simulink model "Plant"  (R2025b)
settings: Solver=VariableStepAuto  StartTime=0.0  StopTime=10.0  RelTol=1e-3
values from neighbouring files (symbols this model uses):
  eul_init = scenario.eul_init    [Brown_6DOF_Init_main.m]    (also in Full_Sim_Init.m; Run_Main.m = runSpec.eul_init)
  g = scenario.g    [Brown_6DOF_Init_main.m]    (also in Full_Sim_Init.m; aircraft_def.m = value)
  J = aircraft.J    [Brown_6DOF_Init_main.m]    (also in Full_Sim_Init.m; HOMEWORK7_trim_linmod_live_source.m = zeros(4,3); aircraft_def.m = I_total)
  Mass = aircraft.Mass    [Brown_6DOF_Init_main.m]    (also in Full_Sim_Init.m; aircraft_def.m = 0)
  omega_init = scenario.omega_init    [Brown_6DOF_Init_main.m]    (also in Full_Sim_Init.m; Run_Main.m = runSpec.omega_init)
  pos_init = scenario.pos_init    [Brown_6DOF_Init_main.m]    (also in Full_Sim_Init.m; Run_Main.m = runSpec.pos_init)
  prop = aircraft.prop    [Brown_6DOF_Init_main.m]    (also in Full_Sim_Init.m; Run_INDI_Qdot_Effectiveness_Audit.m = plant.prop)
  q = q / norm(q)    [HOMEWORK7_trim_linmod_live_source.m]    (also in attitude_complementary_step.m = gyro_meas(2))
  r = positions(i, :).'-cg(:)    [Run_INDI_Qdot_Effectiveness_Audit.m]    (also in attitude_complementary_step.m = gyro_meas(3))
  V_init = scenario.V_init    [Brown_6DOF_Init_main.m]    (also in Full_Sim_Init.m; Run_Main.m = runSpec.V_init)
undefined symbols (not defined in the file or in its folder): F, Light, magnitude, MIL
libraries: eVTOL_lib x23, aerolibwind2 x1
settings Model: Creator=zbrown  LastModifiedBy=zbrown

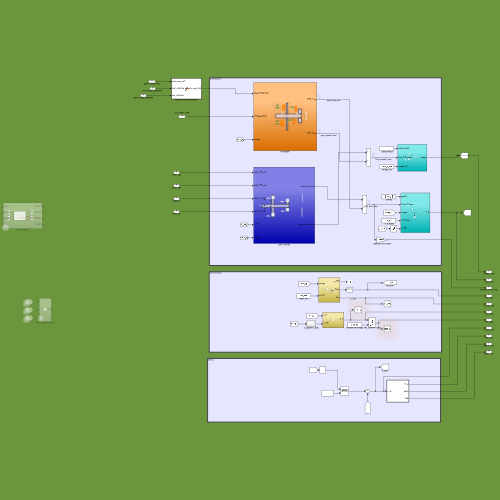
[thumbnail: Simulink's stored preview of the top-level diagram]
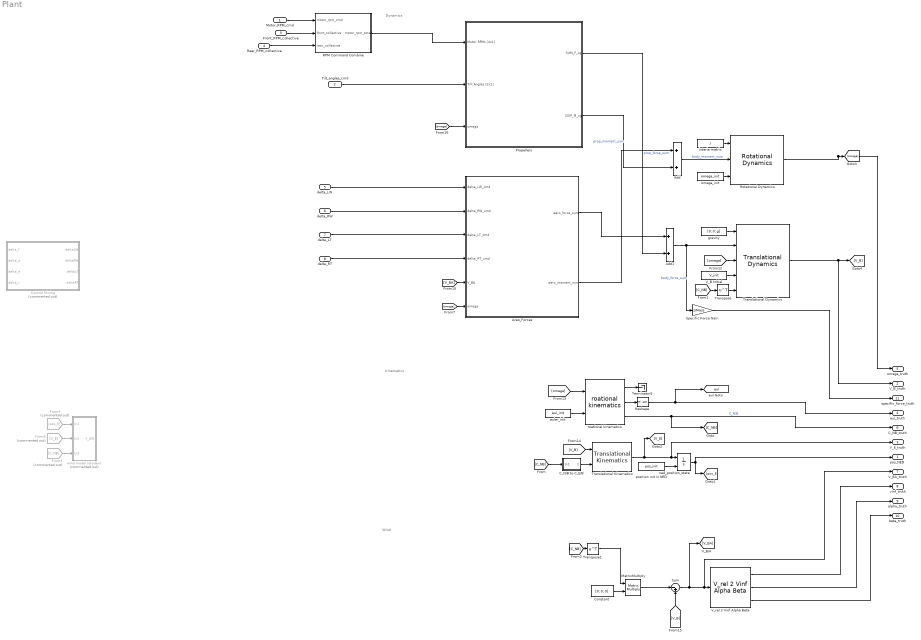
== system Plant ==
  note: Wind
  note: Dynamics
  note: Kinematics
  Motor_RPM_cmd : Inport  PortDimensions=4
  Tilt_angles_cmd : Inport  Port=2  PortDimensions=2
  Front_RPM_collective : Inport  Port=3
  Rear_RPM_collective : Inport  Port=4
  delta_LW : Inport  Port=5
  delta_RW : Inport  Port=6
  delta_LT : Inport  Port=7
  delta_RT : Inport  Port=8
  " V_B Initial" : Constant  Value=V_init
  " gravity" : Constant  Value=[0; 0; g]
  " interia matrix" : Constant  Value=J
  Add : Sum
  Add1 : Sum
  Areo_Forces : Subsystem
  C_N/B to C_E/B : Subsystem
  Constant : Constant  Value=[0; 0; 0]
  Control Mixing : Subsystem  Commented=on
  From3 : From  Commented=on  GotoTag=C_NB
  From4 : From  Commented=on  GotoTag=pos_E
  From5 : From  Commented=on  GotoTag=V_E
  MatrixMultiply : Product  Multiplication=Matrix(*)
  Propellers : Subsystem
  RPM Command Combine : MATLAB Function  TreatAsAtomicUnit=on
  Reshape : Reshape
  Rotational Dynamics : eVTOL_lib/Rotational Dynamics  SystemSampleTime=-1  VariantActivationTime=update diagram  EmptyChoice=off  PassThrough=off  PassThroughVariantControl=(default)  EmptyChoiceVariantControl=(default)  AllowFlexibleInterface=on  Latency=0  AutoFrameSizeCalculation=off
  Specific Force Gain : Gain  Gain=1/Mass
  Sum : Sum  Inputs=|-+
  Terminator5 : Terminator
  Translational Dynamics : eVTOL_lib/Translational Dynamics  SystemSampleTime=-1  VariantActivationTime=update diagram  EmptyChoice=off  PassThrough=off  PassThroughVariantControl=(default)  EmptyChoiceVariantControl=(default)  AllowFlexibleInterface=on  Latency=0  AutoFrameSizeCalculation=off
  Translational Kinematics : eVTOL_lib/Translational Kinematics  SystemSampleTime=-1  VariantActivationTime=update diagram  EmptyChoice=off  PassThrough=off  PassThroughVariantControl=(default)  EmptyChoiceVariantControl=(default)  AllowFlexibleInterface=on  Latency=0  AutoFrameSizeCalculation=off
  Transpose : Math  Operator=transpose
  Transpose1 : Math  Operator=transpose
  V_rel 2 Vinf Alpha Beta : eVTOL_lib/V_rel 2 Vinf Alpha Beta  SystemSampleTime=-1  VariantActivationTime=update diagram  EmptyChoice=off  PassThrough=off  PassThroughVariantControl=(default)  EmptyChoiceVariantControl=(default)  AllowFlexibleInterface=on  Latency=0  AutoFrameSizeCalculation=off
  euler_init : Constant  Value=eul_init
  ned_position_state : Integrator  InitialConditionSource=external
  omega_init : Constant  Value=omega_init
  position init in NED : Constant  Value=pos_init
  roational kinematics : eVTOL_lib/roational kinematics  SystemSampleTime=-1  VariantActivationTime=update diagram  EmptyChoice=off  PassThrough=off  PassThroughVariantControl=(default)  EmptyChoiceVariantControl=(default)  AllowFlexibleInterface=on  Latency=0  AutoFrameSizeCalculation=off
  wind model (dryden) : Subsystem  Commented=on
  pos_NED : Outport
  V_B_truth : Outport  Port=2
  V_E_truth : Outport  Port=3
  eul_truth : Outport  Port=4
  omega_truth : Outport  Port=5
  C_NB_truth : Outport  Port=6
  V_BA_truth : Outport  Port=7
  vinf_truth : Outport  Port=8
  alpha_truth : Outport  Port=9
  beta_truth : Outport  Port=10
  specific_force_truth : Outport  Port=11
  tag scope: eul=global
  wires:
  Transpose/1 -> Translational Dynamics/5
  roational kinematics/3 -> C_NB_truth/1, [C_NB]  "C_N/B"
  roational kinematics/2 -> Reshape/1
  Rotational Dynamics/1 -> omega_truth/1, [omega]
  Translational Dynamics/1 -> [V_B], V_B_truth/1
  Translational Kinematics/1 -> V_E_truth/1, ned_position_state/1, [V_E]
  position init in NED/1 -> ned_position_state/2
  ned_position_state/1 -> [pos_E], pos_NED/1
  euler_init/1 -> roational kinematics/2
  omega_init/1 -> Rotational Dynamics/3
  Add/1 -> Rotational Dynamics/2  "body_moment_sum"
  " interia matrix"/1 -> Rotational Dynamics/1
  " gravity"/1 -> Translational Dynamics/1
  Add1/1 -> Specific Force Gain/1, Translational Dynamics/2  "body_force_sum"
  " V_B Initial"/1 -> Translational Dynamics/4
  Reshape/1 -> eul_truth/1, [eul]
  C_N/B to C_E/B/1(Out1) -> Translational Kinematics/2
  [C_NB] -> C_N/B to C_E/B/1(In1)
  [C_NB] -> Transpose/1
  MatrixMultiply/1 -> Sum/1
  Transpose1/1 -> MatrixMultiply/1
  [C_NB] -> Transpose1/1
  Sum/1 -> V_BA_truth/1, V_rel 2 Vinf Alpha Beta/1, [V_BA]
  From4/1 -> wind model (dryden)/1(In1)
  From5/1 -> wind model (dryden)/2(In2)
  From3/1 -> wind model (dryden)/3(In3)
  V_rel 2 Vinf Alpha Beta/1 -> vinf_truth/1
  V_rel 2 Vinf Alpha Beta/2 -> alpha_truth/1
  V_rel 2 Vinf Alpha Beta/3 -> beta_truth/1
  [omega] -> Translational Dynamics/3
  [omega] -> roational kinematics/1
  [V_B] -> Translational Kinematics/1
  [V_B] -> Sum/2
  Tilt_angles_cmd/1 -> Propellers/2(Tilt Angles [2x1])
  [omega] -> Propellers/3(omega)
  Constant/1 -> MatrixMultiply/2
  Specific Force Gain/1 -> specific_force_truth/1
  Propellers/2(SUM_M_cg) -> Add/2  "prop_moment_sum"
  Propellers/1(SUM_F_cg) -> Add1/2  "prop_force_sum"
  Rear_RPM_collective/1 -> RPM Command Combine/3(rear_collective)
  Motor_RPM_cmd/1 -> RPM Command Combine/1(motor_rpm_cmd)
  Front_RPM_collective/1 -> RPM Command Combine/2(front_collective)
  RPM Command Combine/1(motor_rpm_total) -> Propellers/1(Motor RPMs [4x1])
  delta_LW/1 -> Areo_Forces/1(delta_LW_cmd)
  delta_RW/1 -> Areo_Forces/2(delta_RW_cmd)
  delta_LT/1 -> Areo_Forces/3(delta_LT_cmd)
  delta_RT/1 -> Areo_Forces/4(delta_RT_cmd)
  Areo_Forces/2(aero_moment_sum) -> Add/1
  Areo_Forces/1(aero_force_sum) -> Add1/1
  [V_BA] -> Areo_Forces/5(V_BA)
  [omega] -> Areo_Forces/6(omega)
  roational kinematics/1 -> Terminator5/1

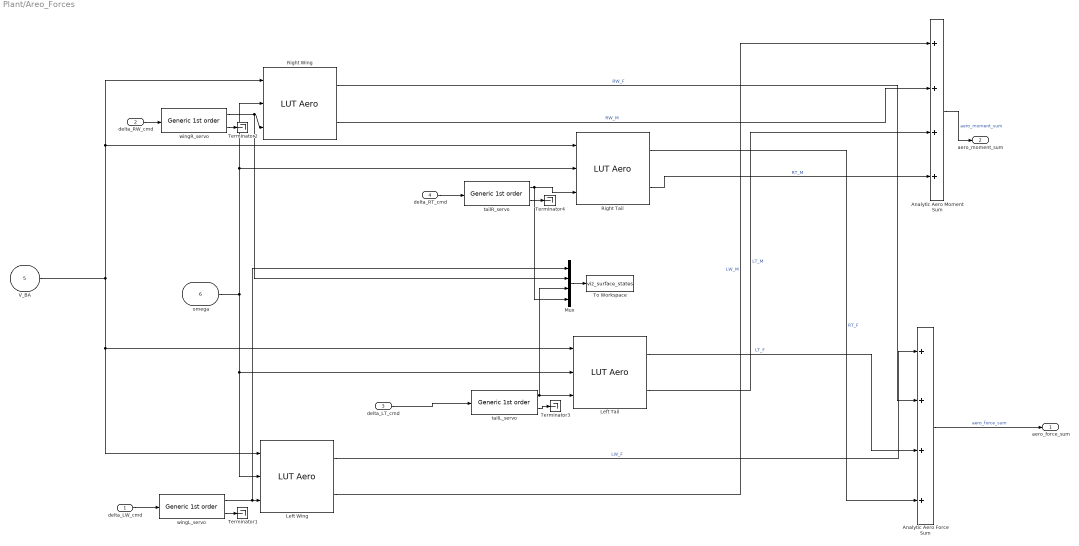
== system Plant/Areo_Forces ==
  delta_LW_cmd : Inport
  delta_RW_cmd : Inport  Port=2
  delta_LT_cmd : Inport  Port=3
  delta_RT_cmd : Inport  Port=4
  V_BA : Inport  Port=5
  omega : Inport  Port=6
  Analytic Aero Force Sum : Sum  Inputs=++++
  Analytic Aero Moment Sum : Sum  Inputs=++++
  Left Tail : eVTOL_lib/LUT Aero  surf=tailL  CG=CG  polar=tailPolar
  Left Wing : eVTOL_lib/LUT Aero  surf=wingL  CG=CG  polar=wingPolar
  Mux : Mux
  Right Tail : eVTOL_lib/LUT Aero  surf=tailR  CG=CG  polar=tailPolar
  Right Wing : eVTOL_lib/LUT Aero  surf=wingR  CG=CG  polar=wingPolar
  Terminator{1..4} (4 alike) : Terminator
  To Workspace : ToWorkspace  VariableName=viz_surface_states  SaveFormat=Structure With Time  SampleTime=-1
  tailL_servo : eVTOL_lib/Generic 1st order  sat_high=tailL.sat_high  sat_low=tailL.sat_low  dot_sat_high=tailL.dot_sat_high  dot_sat_low=tailL.dot_sat_low  init=tailL.init  tau=tailL.tau
  tailR_servo : eVTOL_lib/Generic 1st order  sat_high=tailR.sat_high  sat_low=tailR.sat_low  dot_sat_high=tailR.dot_sat_high  dot_sat_low=tailR.dot_sat_low  init=tailR.init  tau=tailR.tau
  wingL_servo : eVTOL_lib/Generic 1st order  sat_high=wingL.sat_high  sat_low=wingL.sat_low  dot_sat_high=wingL.dot_sat_high  dot_sat_low=wingL.dot_sat_low  init=wingL.init  tau=wingL.tau
  wingR_servo : eVTOL_lib/Generic 1st order  sat_high=wingR.sat_high  sat_low=wingR.sat_low  dot_sat_high=wingR.dot_sat_high  dot_sat_low=wingR.dot_sat_low  init=wingR.init  tau=wingR.tau
  aero_force_sum : Outport
  aero_moment_sum : Outport  Port=2
  wires:
  Analytic Aero Moment Sum/1 -> aero_moment_sum/1  "aero_moment_sum"
  delta_RW_cmd/1 -> wingR_servo/1
  delta_LW_cmd/1 -> wingL_servo/1
  delta_LT_cmd/1 -> tailL_servo/1
  wingL_servo/2 -> Terminator1/1
  Right Wing/1 -> Analytic Aero Force Sum/2  "RW_F"
  omega/1 -> Left Wing/2, Left Tail/2, Right Wing/2, Right Tail/2
  delta_RT_cmd/1 -> tailR_servo/1
  tailR_servo/2 -> Terminator4/1
  Left Wing/2 -> Analytic Aero Moment Sum/1  "LW_M"
  Left Tail/2 -> Analytic Aero Moment Sum/3  "LT_M"
  wingR_servo/1 -> Mux/2, Right Wing/3
  Right Tail/2 -> Analytic Aero Moment Sum/4  "RT_M"
  Right Tail/1 -> Analytic Aero Force Sum/4  "RT_F"
  tailL_servo/2 -> Terminator3/1
  Left Wing/1 -> Analytic Aero Force Sum/1  "LW_F"
  Right Wing/2 -> Analytic Aero Moment Sum/2  "RW_M"
  Left Tail/1 -> Analytic Aero Force Sum/3  "LT_F"
  wingR_servo/2 -> Terminator2/1
  V_BA/1 -> Left Wing/1, Left Tail/1, Right Wing/1, Right Tail/1
  Analytic Aero Force Sum/1 -> aero_force_sum/1  "aero_force_sum"
  wingL_servo/1 -> Mux/1, Left Wing/3
  tailR_servo/1 -> Right Tail/3, Mux/4
  Mux/1 -> To Workspace/1
  tailL_servo/1 -> Mux/3, Left Tail/3

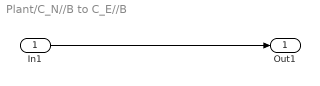
== system Plant/C_N//B to C_E//B ==
  In1 : Inport
  Out1 : Outport
  wires:
  In1/1 -> Out1/1

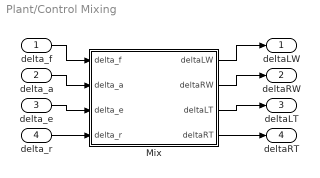
== system Plant/Control Mixing ==
  delta_f : Inport
  delta_a : Inport  Port=2
  delta_e : Inport  Port=3
  delta_r : Inport  Port=4
  Mix : MATLAB Function  TreatAsAtomicUnit=on
  deltaLW : Outport
  deltaRW : Outport  Port=2
  deltaLT : Outport  Port=3
  deltaRT : Outport  Port=4
  wires:
  ? -> ?
  delta_f/1 -> Mix/1(delta_f)
  delta_a/1 -> Mix/2(delta_a)
  delta_e/1 -> Mix/3(delta_e)
  delta_r/1 -> Mix/4(delta_r)
  Mix/1(deltaLW) -> deltaLW/1
  Mix/2(deltaRW) -> deltaRW/1
  Mix/3(deltaLT) -> deltaLT/1
  Mix/4(deltaRT) -> deltaRT/1

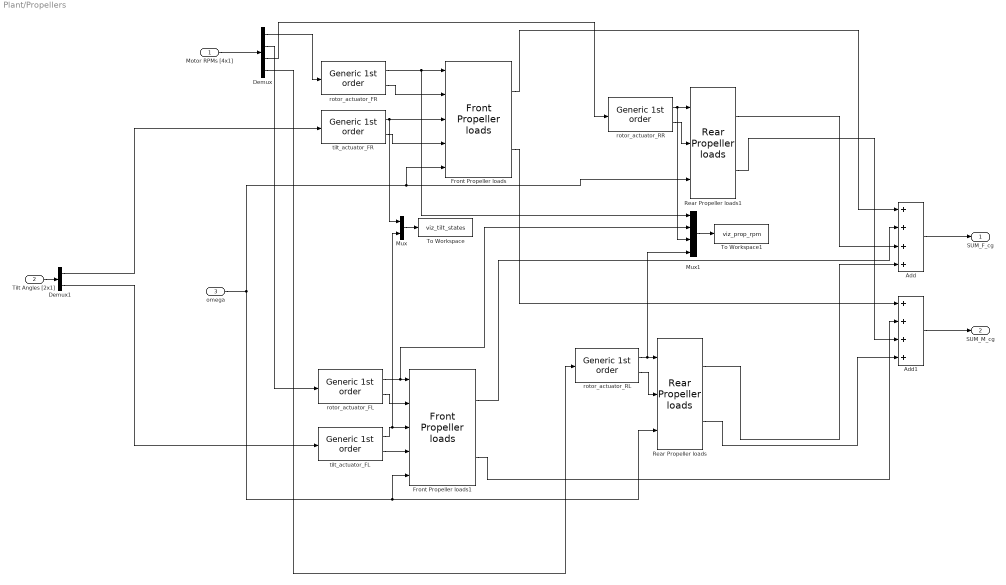
== system Plant/Propellers ==
  Motor RPMs [4x1] : Inport
  Tilt Angles [2x1] : Inport  Port=2
  omega : Inport  Port=3
  Add : Sum  Inputs=++++
  Add1 : Sum  Inputs=++++
  Demux : Demux  Outputs=[1 1 1 1]
  Demux1 : Demux  Outputs=[1 1]
  Front Propeller loads : eVTOL_lib/Front Propeller loads  pivot_pos=prop.posFR  hub_offset=prop.hub_offset  spin_dir=prop.Rspin_dir  kT=prop.k_Thrust  kQ=prop.k_Torque  Jr=prop.Jrotor  CG=CG
  Front Propeller loads1 : eVTOL_lib/Front Propeller loads  pivot_pos=prop.posFL  hub_offset=prop.hub_offset  spin_dir=prop.Lspin_dir  kT=prop.k_Thrust  kQ=prop.k_Torque  Jr=prop.Jrotor  CG=CG
  Mux : Mux  Inputs=2
  Mux1 : Mux
  Rear Propeller loads : eVTOL_lib/Rear Propeller loads  prop_pos=prop.posRL  spin_dir=prop.Lspin_dir  kT=prop.k_Thrust  kQ=prop.k_Torque  Jr=prop.Jrotor  CG=CG
  Rear Propeller loads1 : eVTOL_lib/Rear Propeller loads  prop_pos=prop.posRR  spin_dir=prop.Rspin_dir  kT=prop.k_Thrust  kQ=prop.k_Torque  Jr=prop.Jrotor  CG=CG
  To Workspace : ToWorkspace  VariableName=viz_tilt_states  SaveFormat=Structure With Time  SampleTime=-1
  To Workspace1 : ToWorkspace  VariableName=viz_prop_rpm  SaveFormat=Structure With Time  SampleTime=-1
  rotor_actuator_FL : eVTOL_lib/Generic 1st order  sat_high=prop.rotor.sat_high  sat_low=prop.rotor.sat_low  dot_sat_high=prop.rotor.dot_sat_high  dot_sat_low=prop.rotor.dot_sat_low  init=prop.rotor.init(2)  tau=prop.rotor.tau
  rotor_actuator_FR : eVTOL_lib/Generic 1st order  sat_high=prop.rotor.sat_high  sat_low=prop.rotor.sat_low  dot_sat_high=prop.rotor.dot_sat_high  dot_sat_low=prop.rotor.dot_sat_low  init=prop.rotor.init(1)  tau=prop.rotor.tau
  rotor_actuator_RL : eVTOL_lib/Generic 1st order  sat_high=prop.rotor.sat_high  sat_low=prop.rotor.sat_low  dot_sat_high=prop.rotor.dot_sat_high  dot_sat_low=prop.rotor.dot_sat_low  init=prop.rotor.init(4)  tau=prop.rotor.tau
  rotor_actuator_RR : eVTOL_lib/Generic 1st order  sat_high=prop.rotor.sat_high  sat_low=prop.rotor.sat_low  dot_sat_high=prop.rotor.dot_sat_high  dot_sat_low=prop.rotor.dot_sat_low  init=prop.rotor.init(3)  tau=prop.rotor.tau
  tilt_actuator_FL : eVTOL_lib/Generic 1st order  sat_high=prop.tilt.sat_high  sat_low=prop.tilt.sat_low  dot_sat_high=prop.tilt.dot_sat_high  dot_sat_low=prop.tilt.dot_sat_low  init=prop.tilt.init(2)  tau=prop.tilt.tau
  tilt_actuator_FR : eVTOL_lib/Generic 1st order  sat_high=prop.tilt.sat_high  sat_low=prop.tilt.sat_low  dot_sat_high=prop.tilt.dot_sat_high  dot_sat_low=prop.tilt.dot_sat_low  init=prop.tilt.init(1)  tau=prop.tilt.tau
  SUM_F_cg : Outport
  SUM_M_cg : Outport  Port=2
  wires:
  Add/1 -> SUM_F_cg/1
  Add1/1 -> SUM_M_cg/1
  Motor RPMs [4x1]/1 -> Demux/1
  Tilt Angles [2x1]/1 -> Demux1/1
  omega/1 -> Front Propeller loads/5, Rear Propeller loads1/3, Front Propeller loads1/5, Rear Propeller loads/3
  Front Propeller loads/1 -> Add/1
  Rear Propeller loads1/1 -> Add/3
  Front Propeller loads1/1 -> Add/2
  Rear Propeller loads/1 -> Add/4
  Front Propeller loads/2 -> Add1/1
  Rear Propeller loads1/2 -> Add1/3
  Front Propeller loads1/2 -> Add1/2
  Rear Propeller loads/2 -> Add1/4
  Demux/1 -> rotor_actuator_FR/1
  Demux/2 -> rotor_actuator_FL/1
  Demux/3 -> rotor_actuator_RR/1
  Demux/4 -> rotor_actuator_RL/1
  rotor_actuator_FR/1 -> Mux1/1, Front Propeller loads/1
  rotor_actuator_FR/2 -> Front Propeller loads/2
  tilt_actuator_FR/1 -> Mux/1, Front Propeller loads/3
  tilt_actuator_FR/2 -> Front Propeller loads/4
  Demux1/1 -> tilt_actuator_FR/1
  tilt_actuator_FL/2 -> Front Propeller loads1/4
  rotor_actuator_FL/2 -> Front Propeller loads1/2
  tilt_actuator_FL/1 -> Mux/2, Front Propeller loads1/3
  Demux1/2 -> tilt_actuator_FL/1
  rotor_actuator_RL/2 -> Rear Propeller loads/2
  rotor_actuator_RL/1 -> Mux1/4, Rear Propeller loads/1
  rotor_actuator_RR/2 -> Rear Propeller loads1/2
  rotor_actuator_RR/1 -> Mux1/3, Rear Propeller loads1/1
  Mux/1 -> To Workspace/1
  rotor_actuator_FL/1 -> Mux1/2, Front Propeller loads1/1
  Mux1/1 -> To Workspace1/1

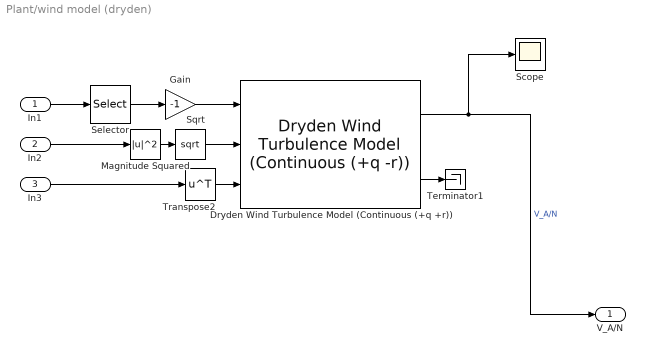
== system Plant/wind model (dryden) ==
  In1 : Inport
  In2 : Inport  Port=2
  In3 : Inport  Port=3
  Dryden Wind Turbulence Model (Continuous (+q +r)) : aerolibwind2/Dryden Wind Turbulence Model  (Continuous (+q -r))  units=Metric (MKS)  spec=MIL-F-8785C  model=Continuous Dryden (+q +r)  W20=15  Wdeg=0  TurbProb=10^-2 - Light  L_high=533.4  Wingspan=10  ts=0.1  Seed=[23341 23342 23343 23344]  T_on=on
      settings: LibrarySourceBlock=|
      | aerolibwind2/Dryden Wind Turbulence Model
      | (Continuous (+q +r))
  Gain : Gain  Gain=-1
  Magnitude Squared : Math  Operator=magnitude^2
  Scope : Scope
  Selector : Selector  InputPortWidth=3  IndexOptions=Index vector (dialog)  Indices=[3]  OutputSizes=1
  Sqrt : Sqrt
  Terminator1 : Terminator
  Transpose2 : Math  Operator=transpose
  V_A/N : Outport
  wires:
  In1/1 -> Selector/1
  Sqrt/1 -> Dryden Wind Turbulence Model (Continuous (+q +r))/2
  Dryden Wind Turbulence Model (Continuous (+q +r))/1 -> V_A/N/1, Scope/1  "V_A/N"
  In3/1 -> Transpose2/1
  Transpose2/1 -> Dryden Wind Turbulence Model (Continuous (+q +r))/3
  In2/1 -> Magnitude Squared/1
  Dryden Wind Turbulence Model (Continuous (+q +r))/2 -> Terminator1/1
  Gain/1 -> Dryden Wind Turbulence Model (Continuous (+q +r))/1
  Selector/1 -> Gain/1
  Magnitude Squared/1 -> Sqrt/1

== matlab function Plant/RPM Command Combine ==
  data: motor_rpm_cmd input; motor_rpm_total output; front_collective input; rear_collective input
function motor_rpm_total = fcn(motor_rpm_cmd, front_collective, rear_collective)
motor_rpm_total = motor_rpm_cmd + [front_collective; front_collective; rear_collective; rear_collective];
end

== matlab function Plant/Control Mixing/Mix ==
  data: delta_f input; deltaLW output; delta_a input; delta_e input; delta_r input; deltaRW output; deltaLT output; deltaRT output
function [deltaLW, deltaRW, deltaLT, deltaRT] = fcn(delta_f, delta_a, delta_e, delta_r)
%#codegen
deltaLW = delta_f + delta_a;
deltaRW = delta_f - delta_a;
deltaLT = delta_e - delta_r;
deltaRT = delta_e + delta_r;
end
